simulink library "sldvlib"  (Simulink 7.6)
settings: Solver=ode45  SolverMode=SingleTasking  StartTime=0.0  StopTime=10.0  RelTol=1e-3
undefined symbols (not defined in the file or in its folder): sldvsubsys
settings Model: Creator=The MathWorks Inc.  ExtModeAutoUpdateStatusClock=off

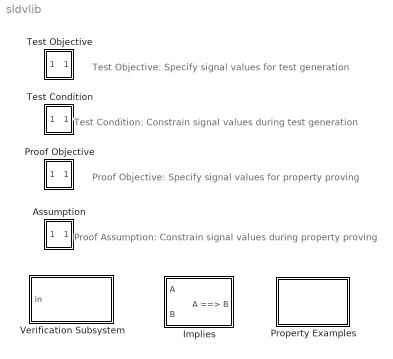
== system sldvlib ==
  note: Test Objective: Specify signal values for
      | test generation
  note: Test Condition: Constrain signal values
      | during test generation
  note: Proof Objective: Specify signal values for
      | property proving
  note: Proof Assumption: Constrain signal values
      | during property proving
  Assumption : Subsystem  mask(Design Verifier Assumption){enabled=on, customAVTBlockType=Assumption, intervals=true, initial=off, dispValues=on, outEnabled=on}
      mask prompts: enabled "Enable"; customAVTBlockType "Type"; intervals "Values"; dispValues "Display values"; outEnabled "Pass through style (show Outport)"
      mask help:
      | Assumes signal values when Simulink Design Verifier proves model properties.  The input signal is assumed to be one of the values listed in the 'Values' parameter.  Two element vectors specify intervals.  Cell arrays specify lists. The signal must match one of the listed values or intervals at every time step.
      | Example Values:
      | true
      | {[0 1], 2, [4 5], 6}
      | {Sldv.Interval(-2, -1), Sldv.Point(0), Sldv.Interval(0, 1, '()'), 1}
      mask init:
      | customAVTParams = customAVTBlock(gcb, 'update_from_mask', intervals);
      settings: AttributesFormatString=%<intervals>
      mask Help: helpview(fullfile(docroot,'toolbox','sldv','sldv.map'),'proofassumption')
      mask StyleString: checkbox,popup(Test Condition|Assumption),edit,checkbox,checkbox,checkbox
      mask CallbackString: ||||customAVTBlock(gcb,'updateDisp');|
      mask Display: image(imread('sldvicon_a_normal.png','BackGroundColor',[1 1 1]),[3 3 19 20]); hide_arrows(true);
  Implies : Subsystem
      mask Type: Design Verifier Implies
      mask Description:
      | Tests whether the first input implies the second.  Outputs false
      | when first input is true and second input is false, otherwise
      | outputs true.
      mask Help: helpview(fullfile(docroot,'toolbox','sldv','sldv.map'),'implies')
      mask Display: disp(' ')
  Proof Objective : Subsystem  mask(Design Verifier Proof Objective){enabled=on, customAVTBlockType=Proof Objective, intervals=true, dispValues=on, outEnabled=on, enableStopSim=off}
      mask prompts: enabled "Enable"; customAVTBlockType "Type"; intervals "Values"; dispValues "Display values"; outEnabled "Pass through style (show Outport)"; enableStopSim "Stop simulation when the property is violated"
      mask help:
      | Proves signal values using Simulink Design Verifier.  The 'Values' parameter specifies input signal values to prove. Two element vectors specify intervals.  Cell arrays specify lists. Signals are proven to satisfy at least one of the values or intervals at every time step.
      | Example Values:
      | true
      | {[0 1], 2, [4 5], 6}
      | {Sldv.Interval(-2, -1), Sldv.Point(0), Sldv.Interval(0, 1, '()'), 1}
      mask init:
      | customAVTParams = customAVTBlock(gcb, 'update_from_mask', intervals);
      settings: AttributesFormatString=%<intervals>
      mask Help: helpview(fullfile(docroot,'toolbox','sldv','sldv.map'),'proofobjective')
      mask StyleString: checkbox,popup(Test Objective|Proof Objective),edit,checkbox,checkbox,checkbox
      mask CallbackString: |||customAVTBlock(gcb,'updateDisp');||
      mask Display: image(imread('sldvicon_p_normal.png','BackGroundColor',[1 1 1]),[3 3 19 20]); hide_arrows(true);
  Property Examples : Subsystem
      settings: OpenFcn=open_system('sldvdemo_properties_spec','force')
      mask Type: Property Examples
      mask Description: These are examples of how to specify properties for proving with Simulink Design Verifier.
      mask Display: disp('Property\nExamples')
  Test Condition : Subsystem  mask(Design Verifier Test Condition){enabled=on, customAVTBlockType=Test Condition, intervals=true, initial=off, dispValues=on, outEnabled=on}
      mask prompts: enabled "Enable"; customAVTBlockType "Type"; intervals "Values"; dispValues "Display values"; outEnabled "Pass through style (show Outport)"
      mask help:
      | Constrains signal values in Simulink Design Verifier test cases. The 'Values' parameter constrains the block input signal.  Two element vectors specify intervals.  Cell arrays specify lists.  The signal must satisfy at least one of the values or intervals at every time step.
      | Example Values:
      | true
      | {[0 1], 2, [4 5], 6}
      | {Sldv.Interval(-2, -1), Sldv.Point(0), Sldv.Interval(0, 1, '()'), 1}
      mask init:
      | customAVTParams = customAVTBlock(gcb, 'update_from_mask', intervals);
      settings: AttributesFormatString=%<intervals>
      mask Help: helpview(fullfile(docroot,'toolbox','sldv','sldv.map'),'testcondition')
      mask StyleString: checkbox,popup(Test Condition|Assumption),edit,checkbox,checkbox,checkbox
      mask CallbackString: ||||customAVTBlock(gcb,'updateDisp');|
      mask Display: image(imread('sldvicon_c_normal.png','BackGroundColor',[1 1 1]),[3 3 19 20]); hide_arrows(true);
  Test Objective : Subsystem  mask(Design Verifier Test Objective){enabled=on, customAVTBlockType=Test Objective, intervals=true, dispValues=on, outEnabled=on}
      mask prompts: enabled "Enable"; customAVTBlockType "Type"; intervals "Values"; dispValues "Display values"; outEnabled "Pass through style (show Outport)"
      mask help:
      | Obtains signal values in Simulink Design Verifier test cases.  The 'Values' parameter specifies the desired input signal values.  Two element vectors specify intervals.  Cell arrays specify lists.  Each list entry might result in a separate test case.
      | Example Values:
      | true
      | {[0 1], 2, [4 5], 6}
      | {Sldv.Interval(-2, -1), Sldv.Point(0), Sldv.Interval(0, 1, '()'), 1}
      mask init:
      | customAVTParams = customAVTBlock(gcb, 'update_from_mask', intervals);
      settings: AttributesFormatString=%<intervals>
      mask Help: helpview(fullfile(docroot,'toolbox','sldv','sldv.map'),'testobjective')
      mask StyleString: checkbox,popup(Test Objective|Proof Objective),edit,checkbox,checkbox
      mask CallbackString: |||customAVTBlock(gcb,'updateDisp');|
      mask Display: image(imread('sldvicon_o_normal.png','BackGroundColor',[1 1 1]),[3 3 19 20]); hide_arrows(true);
  Verification Subsystem : Subsystem  Tag=VerificationSubsystem  Description="Groups Design Verifier blocks into a subsystem whose contents are excluded from the code Real-Time Workshop generates.  This subsystem can include other blocks that compute input signals for the Design Verifier blocks."  DisableCoverage=on  LoadFcn=sldvsubsys('check')  TreatAsAtomicUnit=on  SimViewingDevice=on  mask(VerificationSubsystem){}
      mask init:
      | sldvsubsys('maskInit');
      settings: CopyFcn=sldvsubsys('copy');  OpenFcn=open_system(gcb,'force');
      settings: PreSaveFcn=|
      | set_param(gcb,'SimViewingDevice','on');
      | sldvsubsys('check');
      mask Help: helpview(fullfile(docroot,'toolbox','sldv','sldv.map'),'verificationsubsystem')
      mask Display: image(imread('sldvicon_versubsys.png','BackGroundColor',[1 1 1]),'center');

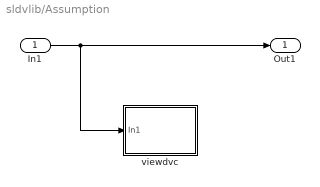
== system sldvlib/Assumption ==
  In1 : Inport
  viewdvc : Subsystem  TreatAsAtomicUnit=on  SimViewingDevice=on  mask(VerificationSubsystem){}
      mask init:
      | sldvsubsys('maskInit');
  Out1 : Outport
  wires:
  In1/1 -> Out1/1, viewdvc/1(In1)

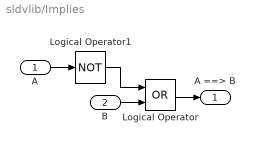
== system sldvlib/Implies ==
  A : Inport
  B : Inport  Port=2
  Logical Operator : Logic  Operator=OR  AllPortsSameDT=off  OutDataTypeStr=boolean
  Logical Operator1 : Logic  Operator=NOT  AllPortsSameDT=off  OutDataTypeStr=boolean
  A ==> B : Outport
  wires:
  B/1 -> Logical Operator/2
  Logical Operator/1 -> A ==> B/1
  A/1 -> Logical Operator1/1
  Logical Operator1/1 -> Logical Operator/1

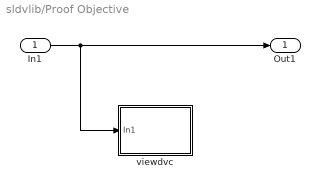
== system sldvlib/Proof Objective ==
  In1 : Inport
  viewdvc : Subsystem  TreatAsAtomicUnit=on  SimViewingDevice=on  mask(VerificationSubsystem){}
      mask init:
      | sldvsubsys('maskInit');
  Out1 : Outport
  wires:
  In1/1 -> Out1/1, viewdvc/1(In1)

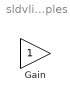
== system sldvlib/Property Examples ==
  Gain : Gain  SaturateOnIntegerOverflow=on  OutDataTypeStr=Inherit: Same as input  ParamDataTypeStr=Inherit: Same as input

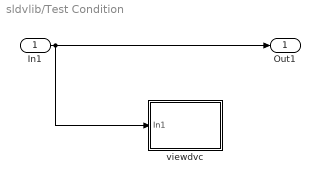
== system sldvlib/Test Condition ==
  In1 : Inport
  viewdvc : Subsystem  TreatAsAtomicUnit=on  SimViewingDevice=on  mask(VerificationSubsystem){}
      mask init:
      | sldvsubsys('maskInit');
  Out1 : Outport
  wires:
  In1/1 -> Out1/1, viewdvc/1(In1)

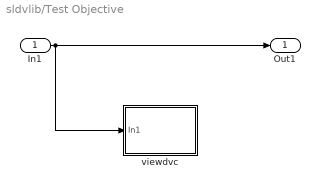
== system sldvlib/Test Objective ==
  In1 : Inport
  viewdvc : Subsystem  TreatAsAtomicUnit=on  SimViewingDevice=on  mask(VerificationSubsystem){}
      mask init:
      | sldvsubsys('maskInit');
  Out1 : Outport
  wires:
  In1/1 -> Out1/1, viewdvc/1(In1)

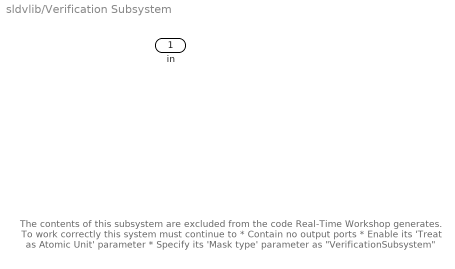
== system sldvlib/Verification Subsystem ==
  note: The contents of this subsystem are excluded from the code Real-Time
      | Workshop generates.
      |
      | To work correctly this system must continue to
      | * Contain no output ports
      | * Enable its 'Treat as Atomic Unit' parameter
      | * Specify its 'Mask type' parameter as "VerificationSubsystem"
  in : Inport

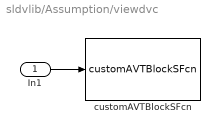
== system sldvlib/Assumption/viewdvc ==
  In1 : Inport
  customAVTBlockSFcn : S-Function  FunctionName=customAVTBlockSFcn  EnableBusSupport=off
  wires:
  In1/1 -> customAVTBlockSFcn/1

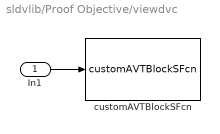
== system sldvlib/Proof Objective/viewdvc ==
  In1 : Inport
  customAVTBlockSFcn : S-Function  FunctionName=customAVTBlockSFcn  EnableBusSupport=off
  wires:
  In1/1 -> customAVTBlockSFcn/1

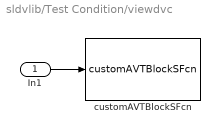
== system sldvlib/Test Condition/viewdvc ==
  In1 : Inport
  customAVTBlockSFcn : S-Function  FunctionName=customAVTBlockSFcn  EnableBusSupport=off
  wires:
  In1/1 -> customAVTBlockSFcn/1

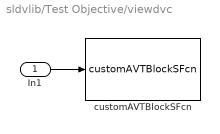
== system sldvlib/Test Objective/viewdvc ==
  In1 : Inport
  customAVTBlockSFcn : S-Function  FunctionName=customAVTBlockSFcn  EnableBusSupport=off
  wires:
  In1/1 -> customAVTBlockSFcn/1
